simulink model "Cyber_Physical_Microgrid"  (R2024b)
settings: Solver=VariableStepAuto  StartTime=0.0  StopTime=270  RelTol=1e-3
values from neighbouring files (symbols this model uses):
  Bat =     [initData.mat]
  droopFC1 = 0.05    [initData.mat]
  droopFC2 = 0.05    [initData.mat]
  droopP2 = 0.05    [initData.mat]
  droopQ1 = 0.05    [initData.mat]
  droopQ2 = 0.05    [initData.mat]
  Pref2 = 0.8    [initData.mat]
  Qref1 = 0    [initData.mat]
  Qref2 = 0    [initData.mat]
  timeACLoadCurtail = 200    [initData.mat]
  timeSolarCurtail = 200    [initData.mat]
  Ts = 5e-05    [initData.mat]
  Ts_AC = 0.0002    [initData.mat]
  Ts_DC = 0.001    [initData.mat]
  volt2 = [270.467186401 250.166401688 246.278575679 243.847178474 242.073246789 240.654489675 239.457734124 238.414696845 237.485238449 236.643553985 235.871256975 235.151075236 ... (161 elements, 1x161)]    [initData.mat]
undefined symbols (not defined in the file or in its folder): BattTempBp, CapLUTBp, CapSOCBp, DiscIntNeverNeededParam, Em, Np, Ns, RInt, Tc_Batt
libraries: nesl_utility x55, fl_lib x52, ee_lib x39, modbuslib x16, spsRMSLib x8, simulink x5, spsFourierLib x2, batteryecm_lib x1, eeTransforms x1
(part 2 of 3)

== system Cyber_Physical_Microgrid/Grid Synchronization ==
  note: breaker command: 1 - islanded (PCC open)
      | 0 - connect to utility (PCC closed)
  note: 1 - start sycnhronisation
      | 0 - stay islanded
  note: microgrid frequency (pu)
  note: utility grid phase angle
  note: microgrid phase angle
  note: new frequency reference sent to
      | microgrid governer
  note: utility grid frequency (pu)
  note: frequency step size (how aggressive we tune frequency)
  Constant1 : Constant  Value=1e-5
  Constant2 : Constant
  Grid Synchronization1 : MATLAB Function  TreatAsAtomicUnit=on
  Step : Step  Time=27  Before=1  After=0  SampleTime=0
  Unit Delay : UnitDelay  InitialCondition=1  SampleTime=Ts_AC  HasFrameUpgradeWarning=on
  Unit Delay1 : UnitDelay  InitialCondition=1  SampleTime=Ts_AC  HasFrameUpgradeWarning=on
  tag scope: freqRef=global, gridEnable=global, synchStart=global
  wires:
  Grid Synchronization1/2(gridEnable) -> Unit Delay/1  "gridEnable"
  Constant1/1 -> Grid Synchronization1/1(deltaF)
  [phiMicro] -> Grid Synchronization1/5(phiMicro)
  Unit Delay1/1 -> [freqRef]
  [freq_gen1_pu] -> Grid Synchronization1/3(freqMicro)
  Grid Synchronization1/1(freqRef) -> Unit Delay1/1
  Constant2/1 -> Grid Synchronization1/2(freqUtility)
  Unit Delay/1 -> [gridEnable]
  [phiUtility] -> Grid Synchronization1/4(phiUtility)
  Step/1 -> [synchStart], Grid Synchronization1/6(synchStart)

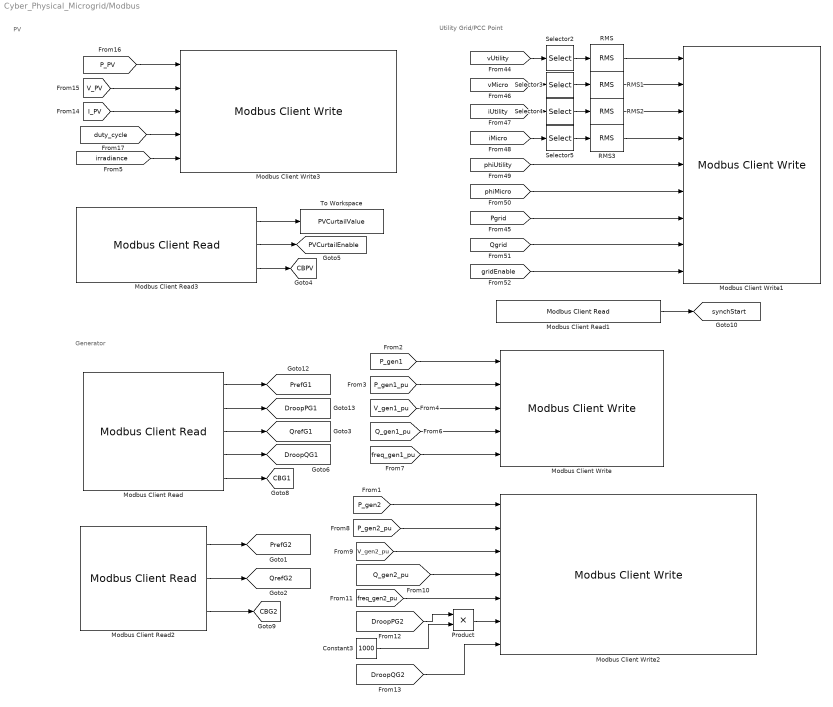
== system Cyber_Physical_Microgrid/Modbus ==
  note: PV
  note: Utility Grid/PCC Point
  note: Generator
  Constant3 : Constant  Value=1000
  Modbus Client Read : modbuslib/Modbus Client Read  RetainClient=gen1  ClientList=gen1  ConnectionEndpoint=192.168.1.202:502  ServerId=1  RegisterTable={ '1', 'PrefG1', '21', 'Holding Register', 'double', '1'; '2', 'DroopPG1', '25', 'Holding Register', 'double', '1'; '3', 'QrefG1', '29', 'Holding Register', 'double', '1'; '4', 'DroopQG1', '34', 'Holding Register', 'double', '1'; '5', 'CBG1', '38', 'Coil', 'bit', '1' }  SampleTime=1
  Modbus Client Read1 : modbuslib/Modbus Client Read  RetainClient=ModbusClient  ClientList=ModbusClient  ConnectionEndpoint=192.168.1.201:502  ServerId=1  RegisterTable={ '1', 'synchStart', '38', 'Coil', 'bit', '1' }  SampleTime=1
  Modbus Client Read2 : modbuslib/Modbus Client Read  RetainClient=gen2  ClientList=gen2  ConnectionEndpoint=192.168.1.203:502  ServerId=1  RegisterTable={ '1', 'PrefG2', '21', 'Holding Register', 'double', '1'; '2', 'QrefG2', '29', 'Holding Register', 'double', '1'; '3', 'CBG2', '38', 'Coil', 'bit', '1' }  SampleTime=1
  Modbus Client Read3 : modbuslib/Modbus Client Read  RetainClient=pv  ClientList=pv  ConnectionEndpoint=192.168.1.204:502  ServerId=1  RegisterTable={ '1', 'PvCurtailValue', '21', 'Holding Register', 'double', '1'; '2', 'curtail enable', '25', 'Coil', 'bit', '1'; '3', 'CBPV', '29', 'Coil', 'bit', '1' }  SampleTime=1
  Modbus Client Write : modbuslib/Modbus Client Write  RetainClient=gen1  ClientList=gen1  ConnectionEndpoint=192.168.1.202:502  ServerId=1  RegisterTable={ '1', 'P_gen1', '1', 'Holding Register', 'double'; '2', 'P_gen1_pu', '5', 'Holding Register', 'double'; '3', 'V_gen1_pu', '9', 'Holding Register', 'double'; '4', 'Q_gen1_pu', '13', 'Holding Register', 'double'; '5', 'freq_gen1_pu', '17', 'Holding Register', 'double' }  SampleTime=1
  Modbus Client Write1 : modbuslib/Modbus Client Write  RetainClient=ModbusClient  ClientList=ModbusClient  ConnectionEndpoint=192.168.1.201:502  ServerId=1  RegisterTable={ '1', 'vUtility_rms', '1', 'Holding Register', 'double'; '2', 'vMicro_rms', '5', 'Holding Register', 'double'; '3', 'iUtility_rms', '9', 'Holding Register', 'double'; '4', 'iMicro_rms', '13', 'Holding Register', 'double'; '5', 'phiUtility', '17', 'Holding Register', 'double'; '6', 'phiMicro', '21', 'Holding Register', 'double'; '7', 'Pgrid', '25', 'Holding Register', 'double'; '8', 'Qgrid', '29', 'Holding Register', 'double'; '9', 'gridEnable', '34', 'Coil', 'bit' }  SampleTime=1
  Modbus Client Write2 : modbuslib/Modbus Client Write  RetainClient=gen2  ClientList=gen2  ConnectionEndpoint=192.168.1.203:502  ServerId=1  RegisterTable={ '1', 'P_gen2', '1', 'Holding Register', 'double'; '2', 'P_gen2_pu', '5', 'Holding Register', 'double'; '3', 'V_gen2_pu', '9', 'Holding Register', 'double'; '4', 'Q_gen2_pu', '13', 'Holding Register', 'double'; '5', 'freq_gen2_pu', '17', 'Holding Register', 'double'; '6', 'DroopPG2', '25', 'Holding Register', 'double'; '7', 'DroopQG2', '34', 'Holding Register', 'double' }  SampleTime=1
  Modbus Client Write3 : modbuslib/Modbus Client Write  RetainClient=pv  ClientList=pv  ConnectionEndpoint=192.168.1.204:502  ServerId=1  RegisterTable={ '1', 'P_PV', '1', 'Holding Register', 'double'; '2', 'V_PV', '5', 'Holding Register', 'double'; '3', 'I_PV', '9', 'Holding Register', 'double'; '4', 'duty cycle', '13', 'Holding Register', 'double'; '5', 'irradiance', '17', 'Holding Register', 'double' }  SampleTime=1
  Product : Product
  RMS{,1..3} (4 alike) : spsRMSLib/RMS  TrueRMS=on  Freq=50  RMSInit=120  Ts=0
  Selector{2..5} (4 alike) : Selector  InputPortWidth=3  IndexOptions=Index vector (dialog)  Indices=1  OutputSizes=1
  To Workspace : ToWorkspace  VariableName=PVCurtailValue  SaveFormat=Timeseries  SampleTime=-1
  tag scope: CBG1=global, CBG2=global, CBPV=global, DroopPG1=global, DroopQG1=global, PVCurtailEnable=global, PrefG1=global, PrefG2=global, QrefG1=global, QrefG2=global, synchStart=global
  wires:
  [V_gen1_pu] -> Modbus Client Write/3
  [P_gen1_pu] -> Modbus Client Write/2
  Modbus Client Read/1 -> [PrefG1]
  [P_gen1] -> Modbus Client Write/1
  [freq_gen1_pu] -> Modbus Client Write/5
  [Q_gen1_pu] -> Modbus Client Write/4
  Modbus Client Read/2 -> [DroopPG1]
  Modbus Client Read/5 -> [CBG1]
  [iMicro] -> Selector5/1
  RMS2/1 -> Modbus Client Write1/3
  RMS/1 -> Modbus Client Write1/1
  RMS3/1 -> Modbus Client Write1/4
  [iUtility] -> Selector4/1
  [phiUtility] -> Modbus Client Write1/5
  [Qgrid] -> Modbus Client Write1/8
  [Pgrid] -> Modbus Client Write1/7
  Selector4/1 -> RMS2/1
  Selector5/1 -> RMS3/1
  RMS1/1 -> Modbus Client Write1/2
  Modbus Client Read1/1 -> [synchStart]
  [vMicro] -> Selector3/1
  [vUtility] -> Selector2/1
  [phiMicro] -> Modbus Client Write1/6
  [gridEnable] -> Modbus Client Write1/9
  Selector2/1 -> RMS/1
  Selector3/1 -> RMS1/1
  Constant3/1 -> Product/2
  [P_gen2] -> Modbus Client Write2/1
  [DroopPG2] -> Product/1
  [V_gen2_pu] -> Modbus Client Write2/3
  Product/1 -> Modbus Client Write2/6
  Modbus Client Read2/3 -> [CBG2]
  Modbus Client Read2/2 -> [QrefG2]
  [DroopQG2] -> Modbus Client Write2/7
  [freq_gen2_pu] -> Modbus Client Write2/5
  [Q_gen2_pu] -> Modbus Client Write2/4
  [P_gen2_pu] -> Modbus Client Write2/2
  Modbus Client Read2/1 -> [PrefG2]
  Modbus Client Read3/3 -> [CBPV]
  [P_PV] -> Modbus Client Write3/1
  Modbus Client Read3/1 -> To Workspace/1
  [irradiance] -> Modbus Client Write3/5
  [duty_cycle] -> Modbus Client Write3/4
  [I_PV] -> Modbus Client Write3/3
  Modbus Client Read3/2 -> [PVCurtailEnable]
  [V_PV] -> Modbus Client Write3/2
  Modbus Client Read/3 -> [QrefG1]
  Modbus Client Read/4 -> [DroopQG1]

== system Cyber_Physical_Microgrid/PQ meas ==
  PS-Simulink Converter : nesl_utility/PS-Simulink Converter  PhysicalDomain=network_engine_domain  SubClassName=ps_output  LeftPortType=input  RightPortType=output  PseudoPeriodic=off  Frequencies=[]  VectorFormat=1-D array  Unit=W  AffineConversion=off
  PS-Simulink Converter1 : nesl_utility/PS-Simulink Converter  PhysicalDomain=network_engine_domain  SubClassName=ps_output  LeftPortType=input  RightPortType=output  PseudoPeriodic=off  Frequencies=[]  VectorFormat=1-D array  Unit=V*A  AffineConversion=off
  Power Sensor (Three-Phase) : ee_lib/Sensors & Transducers/Power Sensor (Three-Phase)  load_type=ee.enum.passive.type_balanced.balanced  f0=50 Hz
      settings: InternalSimscapePortConfiguration="{\"Bottom\":[],\"Left\":[{\"id\":\"N1\",\"label\":\"~1\",\"type\":\"foundation.electrical.three_phase\"}],\"Right\":[{\"id\":\"N2\",\"label\":\"~2\",\"type\":\"foundation.electrical.three_phase\"}],\"Top\":[{\"id\":\"Pm\",\"label\":\"P\",\"type\":\"output\"},{\"id\":\"Qm\",\"label\":\"Q\",\"type\":\"output\"}]}"
  Subsystem : Subsystem
  Subsystem1 : Subsystem
  ~1 : PMIOPort  Side=Left
  ~2 : PMIOPort  Port=2  Side=Right
  tag scope: P_load=global, Q_load=global
  wires:
  PS-Simulink Converter1/1 -> Subsystem1/1(In1)
  Subsystem1/1(Out1) -> [Q_load]  "Q_load"
  Subsystem/1(Out1) -> [P_load]  "P_load"
  PS-Simulink Converter/1 -> Subsystem/1(In1)
  connections:
  ~2/RConn1 -- Power Sensor (Three-Phase)/RConn1
  Power Sensor (Three-Phase)/LConn1 -- ~1/RConn1
  PS-Simulink Converter/LConn1 -- Power Sensor (Three-Phase)/LConn2
  PS-Simulink Converter1/LConn1 -- Power Sensor (Three-Phase)/LConn3

== system Cyber_Physical_Microgrid/PV Array ==
  Display : Display
  ERef : fl_lib/Electrical/Electrical Elements/Electrical Reference
  Product1 : Product
  Repeating Sequence Interpolated : simulink/Sources/Repeating Sequence Interpolated  OutValues=[1e-3 1e-3 1 1]*1000  TimeValues=[0 1 5 300]  LookUpMeth=Interpolation-Use End Values  tsamp=Ts_DC  OutMin=[]  OutMax=[]  OutDataTypeStr=double  OutputDataTypeScalingMode=double  OutDataType=fixdt(0,8)  OutScaling=2^-10
  Sensing Current : Subsystem
      settings: PortSchema="{\"entries\":[{\"content\":{\"sides\":[{\"content\":{\"connectorIds\":[\"LConn1\"]},\"type\":\"ConnectorPlacement.EquallySpacedRectSide\",\"uuid\":\"08eaf192-3836-4d70-9f6a-c3aee0977ea6\"},{\"content\":{\"connectorIds\":[\"RConn1\"],\"side\":\"RIGHT\"},\"type\":\"ConnectorPlacement.EquallySpacedRectSide\",\"uuid\":\"69615d36-c1bf-4d31-b3e4-77c73286e7c7\"},{\"content\":{\"connectorIds\":[\"Out1\"],\"side\":\"TOP\"},\"type\":\"ConnectorPlacement.EquallySpacedRectSide\",\"uuid\":\"21e31d90-f675-47e5-98f5-1bf7e6a5fdbe\"}]},\"type\":\"ConnectorPlacement.EquallySpacedConnector\",\"uuid\":\"068abd2e-abc9-41d7-b40e-d83d3e3b9346\"}],\"packageUris\":[\"http://schema.mathworks.com/mf0/Connector/R2020b\"],\"version\":\"1.0\"}"
      mask Display: disp('i')
  Simulink-PS Converter : nesl_utility/Simulink-PS Converter  PhysicalDomain=network_engine_domain  SubClassName=ps_input  LeftPortType=input  RightPortType=output  PseudoPeriodic=off  Frequencies=[]  NoiseDistribution=none  NoiseParameters=[]  Unit=1  AffineConversion=off  FilteringAndDerivatives=provide  SimscapeFilterOrder=1  InputFilterTimeConstant=0.001  UdotUserProvided=0
  Solar Cell : ee_lib/Sources/Solar Cell  PartSpecification="{\"DatasetId\":\"Amerisolar|AS_6M30_HC_320W|simscape.electrical.solarCell\",\"DisplayName\":\"Amerisolar:AS_6M30_HC_320W\"}"  prm=3  Isc=10.14 A  Voc=0.67 V  Is=3.24823447983853e-07 A  Is2=9.37081970792037e-10 A  Iph=10.140005507508 A  Ir0=1000 W/m^2  ec=1.51118472243322  N2=2.60259908345858  Rs=1.94548269975201e-05 Ohm  Rp=682.95993142779 Ohm  N_series=60*100  N_parallel=30  TIPH1=0.000499942933005141 1/K  EG=1.12 eV  TXIS1=4.23641510120988  TXIS2=16.2689137700667  TRS1=0.243341028305912  TRP1=0 % Parameter not set  Tmeas=25 degC  TFIXED=30 degC  thermal_mass=100 % Parameter not set J/K  initial_temperature=25 degC
      settings: AttributesFormatString=Amerisolar:AS_6M30_HC_320W
  Terminator : Terminator
  sensing voltage : Subsystem
      settings: PortSchema="{\"entries\":[{\"content\":{\"sides\":[{\"content\":{\"connectorIds\":[\"LConn1\"]},\"type\":\"ConnectorPlacement.EquallySpacedRectSide\",\"uuid\":\"08eaf192-3836-4d70-9f6a-c3aee0977ea6\"},{\"content\":{\"connectorIds\":[\"RConn1\"],\"side\":\"RIGHT\"},\"type\":\"ConnectorPlacement.EquallySpacedRectSide\",\"uuid\":\"69615d36-c1bf-4d31-b3e4-77c73286e7c7\"},{\"content\":{\"connectorIds\":[],\"side\":\"TOP\"},\"type\":\"ConnectorPlacement.EquallySpacedRectSide\",\"uuid\":\"21e31d90-f675-47e5-98f5-1bf7e6a5fdbe\"},{\"content\":{\"connectorIds\":[\"Out1\"],\"side\":\"BOTTOM\"},\"type\":\"ConnectorPlacement.EquallySpacedRectSide\",\"uuid\":\"23a77980-6beb-4147-b48e-adf9e1983263\"}]},\"type\":\"ConnectorPlacement.EquallySpacedConnector\",\"uuid\":\"068abd2e-abc9-41d7-b40e-d83d3e3b9346\"}],\"packageUris\":[\"http://schema.mathworks.com/mf0/Connector/R2020b\"],\"version\":\"1.0\"}"
      mask Display: disp('v')
  - : PMIOPort  Side=Left
  -1 : PMIOPort  Port=2  Side=Left
  tag scope: I_PV=global, V_PV=global, irradiance=global
  wires:
  sensing voltage/1(V) -> Display/1, [V_PV], Product1/2  "V_PV"
  Product1/1 -> Terminator/1  "P_PV"
  Repeating Sequence Interpolated/1 -> [irradiance], Simulink-PS Converter/1  "irradiance"
  Sensing Current/1(I) -> [I_PV], Product1/1  "I_PV"
  connections:
  Solar Cell/LConn1 -- Simulink-PS Converter/RConn1
  Solar Cell/LConn2 -- Sensing Current/LConn1
  sensing voltage/RConn1 -- Solar Cell/RConn1 -- ERef/LConn1 -- -1/RConn1
  sensing voltage/LConn1 -- -/RConn1 -- Sensing Current/RConn1

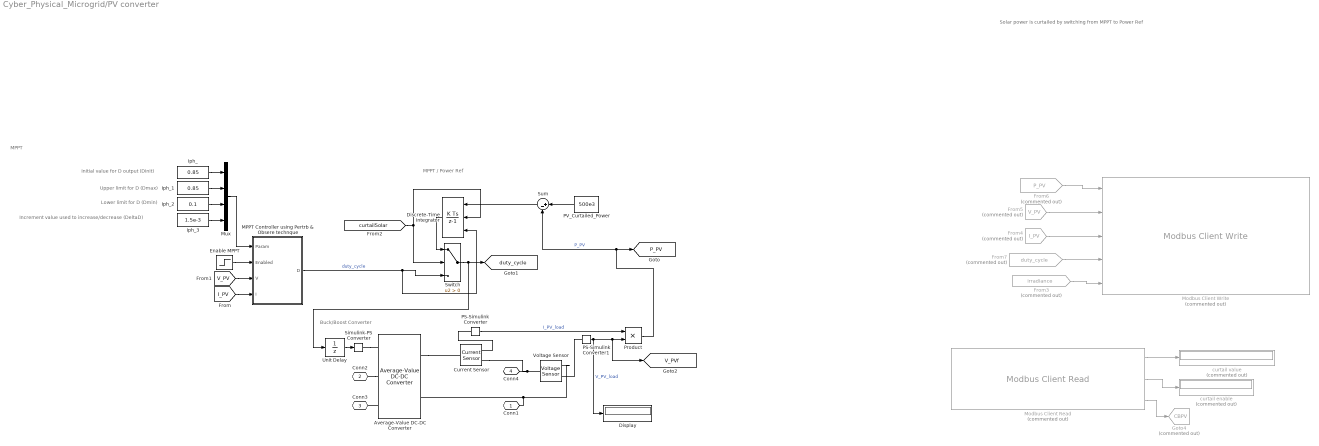
== system Cyber_Physical_Microgrid/PV converter ==
  note: Lower limit for D (Dmin)
  note: Upper limit for D (Dmax)
  note: Increment value used to increase/decrease (DeltaD)
  note: Initial value for D output (Dinit)
  note: Solar power is curtailed by switching from MPPT to Power Ref
  note: MPPT / Power Ref
  note: MPPT
  note: Buck/Boost Converter
  Average-Value DC-DC Converter : ee_lib/Semiconductors & Converters/Converters/Average-Value DC-DC Converter  control_option=ee.enum.converters.controlinput.dutycycle  converter_type=ee.enum.converters.dcdctype.buckboost  efficiency_option=ee.enum.converters.efficiency.constant  efficiency_fixed=100  i_vec=[0, 2, 5] A  efficiency_vec=[90, 95, 98]
      settings: InternalSimscapePortConfiguration="{\"Bottom\":[],\"Left\":[{\"id\":\"DutyCycle\",\"label\":\"DutyCycle\",\"type\":\"input\"},{\"id\":\"p1\",\"label\":\"1+\",\"type\":\"foundation.electrical.electrical\"},{\"id\":\"n1\",\"label\":\"1-\",\"type\":\"foundation.electrical.electrical\"}],\"Right\":[{\"id\":\"p2\",\"label\":\"2+\",\"type\":\"foundation.electrical.electrical\"},{\"id\":\"n2\",\"label\":\"2-\",\"type\":\"foundation.electrical.electrical\"}],\"Top\":[]}"
  Current Sensor : fl_lib/Electrical/Electrical Sensors/Current Sensor
  Discrete-Time Integrator : DiscreteIntegrator  gainval=1e-6  ExternalReset=rising  InitialConditionSource=external  SampleTime=-1  ICPrevOutput=DiscIntNeverNeededParam  ICPrevScaledInput=DiscIntNeverNeededParam
  Display : Display
  Enable MPPT : Step  Time=0.1  SampleTime=Ts_DC
  From3 : From  Commented=on  GotoTag=irradiance  TagVisibility=global
  From4 : From  Commented=on  GotoTag=I_PV  TagVisibility=global
  From5 : From  Commented=on  GotoTag=V_PV  TagVisibility=global
  From6 : From  Commented=on  GotoTag=P_PV  TagVisibility=global
  From7 : From  Commented=on  GotoTag=duty_cycle  TagVisibility=global
  Goto4 : Goto  Commented=on  GotoTag=CBPV  TagVisibility=global
  Iph_ : Constant  Value=0.85  SampleTime=Ts_DC
  Iph_1 : Constant  Value=0.85  SampleTime=Ts_DC
  Iph_2 : Constant  Value=0.1  SampleTime=Ts_DC
  Iph_3 : Constant  Value=1.5e-3  SampleTime=Ts_DC
  "MPPT Controller using Pertrb & Obsere technque " : MATLAB Function  SystemSampleTime=Ts
  Modbus Client Read : modbuslib/Modbus Client Read  Commented=on  RetainClient=No Modbus client available  ClientList=No Modbus client available  ConnectionEndpoint=No Modbus client selected  ServerId=1  RegisterTable={ '1', 'PvCurtailValue', '21', 'Holding Register', 'double', '1'; '2', 'curtail enable', '25', 'Coil', 'bit', '1'; '3', 'CBPV', '29', 'Coil', 'bit', '1' }  SampleTime=1
  Modbus Client Write : modbuslib/Modbus Client Write  Commented=on  RetainClient=No Modbus client available  ClientList=No Modbus client available  ConnectionEndpoint=No Modbus client selected  ServerId=1  RegisterTable={ '1', 'P_PV', '1', 'Holding Register', 'double'; '2', 'V_PV', '5', 'Holding Register', 'double'; '3', 'I_PV', '9', 'Holding Register', 'double'; '4', 'duty cycle', '13', 'Holding Register', 'double'; '5', 'irradiance', '17', 'Holding Register', 'double' }  SampleTime=1
  Mux : Mux
  PS-Simulink Converter : nesl_utility/PS-Simulink Converter  PhysicalDomain=network_engine_domain  SubClassName=ps_output  LeftPortType=input  RightPortType=output  PseudoPeriodic=off  Frequencies=[]  VectorFormat=1-D array  Unit=inherit  AffineConversion=off
  PS-Simulink Converter1 : nesl_utility/PS-Simulink Converter  PhysicalDomain=network_engine_domain  SubClassName=ps_output  LeftPortType=input  RightPortType=output  PseudoPeriodic=off  Frequencies=[]  VectorFormat=1-D array  Unit=inherit  AffineConversion=off
  PV_Curtailed_Power : Constant  Value=500e3
  Product : Product
  Simulink-PS Converter : nesl_utility/Simulink-PS Converter  PhysicalDomain=network_engine_domain  SubClassName=ps_input  LeftPortType=input  RightPortType=output  PseudoPeriodic=off  Frequencies=[]  NoiseDistribution=none  NoiseParameters=[]  Unit=1  AffineConversion=off  FilteringAndDerivatives=provide  SimscapeFilterOrder=1  InputFilterTimeConstant=0.001  UdotUserProvided=0
  Sum : Sum  Inputs=|+-
  Switch : Switch  Criteria=u2 > Threshold  SaturateOnIntegerOverflow=off  InputSameDT=off
  Unit Delay : UnitDelay  InitialCondition=0.99  SampleTime=-1  HasFrameUpgradeWarning=on
  Voltage Sensor : fl_lib/Electrical/Electrical Sensors/Voltage Sensor
  curtail enable : Display  Commented=on
      settings: Format=decimal (Stored Integer)  Decimation=4
  curtail value : Display  Commented=on
      settings: Format=decimal (Stored Integer)  Decimation=4
  Conn1 : PMIOPort  Side=Left
  Conn2 : PMIOPort  Port=2  Side=Left
  Conn3 : PMIOPort  Port=3  Side=Left
  Conn4 : PMIOPort  Port=4  Side=Left
  tag scope: P_PV=global, V_PVf=global, duty_cycle=global
  wires:
  From7/1 -> Modbus Client Write/4
  Enable MPPT/1 -> "MPPT Controller using Pertrb & Obsere technque "/2(Enabled)
  Modbus Client Read/2 -> curtail enable/1
  Iph_1/1 -> Mux/2
  Mux/1 -> "MPPT Controller using Pertrb & Obsere technque "/1(Param)
  [V_PV] -> "MPPT Controller using Pertrb & Obsere technque "/3(V)
  Unit Delay/1 -> Simulink-PS Converter/1
  From4/1 -> Modbus Client Write/3
  Iph_2/1 -> Mux/3
  PS-Simulink Converter1/1 -> Display/1, [V_PVf], Product/2  "V_PV_load"
  [curtailSolar] -> Discrete-Time Integrator/2, Switch/2
  Iph_/1 -> Mux/1
  From5/1 -> Modbus Client Write/2
  PS-Simulink Converter/1 -> Product/1  "I_PV_load"
  Iph_3/1 -> Mux/4
  From6/1 -> Modbus Client Write/1
  Sum/1 -> Discrete-Time Integrator/1
  Modbus Client Read/3 -> Goto4/1
  "MPPT Controller using Pertrb & Obsere technque "/1(D) -> Discrete-Time Integrator/3, Switch/3  "duty_cycle"
  PV_Curtailed_Power/1 -> Sum/1
  Modbus Client Read/1 -> curtail value/1
  Product/1 -> Sum/2, [P_PV]  "P_PV"
  From3/1 -> Modbus Client Write/5
  [I_PV] -> "MPPT Controller using Pertrb & Obsere technque "/4(I)
  Discrete-Time Integrator/1 -> Switch/1
  Switch/1 -> Unit Delay/1, [duty_cycle]
  connections:
  Conn2/RConn1 -- Average-Value DC-DC Converter/LConn2
  Current Sensor/RConn2 -- Voltage Sensor/LConn1 -- Conn4/RConn1
  Simulink-PS Converter/RConn1 -- Average-Value DC-DC Converter/LConn1
  Average-Value DC-DC Converter/RConn1 -- Current Sensor/LConn1
  Voltage Sensor/RConn2 -- Conn1/RConn1 -- Average-Value DC-DC Converter/RConn2
  PS-Simulink Converter/LConn1 -- Current Sensor/RConn1
  Average-Value DC-DC Converter/LConn3 -- Conn3/RConn1
  PS-Simulink Converter1/LConn1 -- Voltage Sensor/RConn1

== system Cyber_Physical_Microgrid/Power Converter ==
  AC/DC Power Conversion : Subsystem
      settings: PortSchema="{\"entries\":[{\"content\":{\"sides\":[{\"content\":{\"connectorIds\":[\"LConn1\"]},\"type\":\"ConnectorPlacement.EquallySpacedRectSide\",\"uuid\":\"019ca52f-1b20-4f8a-8000-26047d27ba44\"},{\"content\":{\"connectorIds\":[\"RConn1\",\"RConn2\"],\"side\":\"RIGHT\"},\"type\":\"ConnectorPlacement.EquallySpacedRectSide\",\"uuid\":\"bc0710a3-2fa6-4c07-a357-204360cbd971\"},{\"content\":{\"connectorIds\":[\"In1\",\"In2\"],\"side\":\"TOP\"},\"type\":\"ConnectorPlacement.EquallySpacedRectSide\",\"uuid\":\"62c22250-eba7-4d66-a03a-98d0551949f6\"}]},\"type\":\"ConnectorPlacement.EquallySpacedConnector\",\"uuid\":\"4a6536c9-62d3-4a93-9f4d-cdcce83d66f7\"}],\"packageUris\":[\"http://schema.mathworks.com/mf0/Connector/R2020b\"],\"version\":\"1.0\"}"
      mask Display: disp('Ideal AC/DC\nPower Conversion')
  Current Sensor : fl_lib/Electrical/Electrical Sensors/Current Sensor
  Display : Display
  Electrical Reference : fl_lib/Electrical/Electrical Elements/Electrical Reference
  PS-Simulink Converter : nesl_utility/PS-Simulink Converter  PhysicalDomain=network_engine_domain  SubClassName=ps_output  LeftPortType=input  RightPortType=output  PseudoPeriodic=off  Frequencies=[]  VectorFormat=inherit  Unit=inherit  AffineConversion=off
  PS-Simulink Converter1 : nesl_utility/PS-Simulink Converter  PhysicalDomain=network_engine_domain  SubClassName=ps_output  LeftPortType=input  RightPortType=output  PseudoPeriodic=off  Frequencies=[]  VectorFormat=inherit  Unit=inherit  AffineConversion=off
  Product : Product
  Qref : simulink/Sources/Repeating Sequence Interpolated  OutValues=[0 0 0 0]*1e5  TimeValues=[0 11 13 50]  LookUpMeth=Interpolation-Use End Values  tsamp=Ts_AC  OutMin=[]  OutMax=[]  OutDataTypeStr=double  OutputDataTypeScalingMode=double  OutDataType=fixdt(0,8)  OutScaling=2^-10
  Solver Configuration : nesl_utility/Solver Configuration  PhysicalDomain=network_engine_domain  SubClassName=solver  LeftPortType=input  RightPortType=generic  Tones=[]  Harmonics=[]  SimulateNoise=off  Profile=off  UseLocalSampling=off  EnableSwitchedLinearOptims=on  FrequencyDomain=off  UseCCode=off  RelTol=0.001  AbsTol=1e-06  MinStep=1e-09  ToWorkspace=off  RevertToSquareIcSolve=off  NumHomotopyIterations=100  PhasorMode=off  PhasorModeNumHarmonics=1  ConsistencySolver=NEWTON_FTOL  IndexReductionMethod=DerivativeReplacement  DoDC=off  ResidualTolerance=1e-09  ConsistencyTolSource=GLOBAL  ConsistencyAbsTol=0.001  ConsistencyRelTol=0.001  ConsistencyTolFactor=0.001  UseLocalSolver=on  LocalSolverChoice=NE_PARTITIONING_ADVANCER  ResolveIndetEquations=on  FunctionEvalNumThread=1  LocalSolverSampleTime=Ts_DC  DoFixedCost=on  MaxNonlinIter=1  MaxModeIter=2  ComputeImpulses=off  ImpulseIterations=2  LinearAlgebra=auto  LinearAlgebraNumThread=0  EquationFormulation=NE_TIME_EF  DelaysMemoryBudget=1024  AutomaticFiltering=on  FilteringTimeConstant=0.001  PartitionStorageMethod=AS_NEEDED  PartitionMemoryBudget=1024  PartitionMethod=ROBUST  MultibodyUseLocalSolver=off  MultibodyLocalSolverChoice=ODE1  MultibodyLocalSolverSampleTime=0.001
  Voltage Sensor : fl_lib/Electrical/Electrical Sensors/Voltage Sensor
  ~ : PMIOPort  Side=Left
  + : PMIOPort  Port=2  Side=Right
  - : PMIOPort  Port=3  Side=Right
  wires:
  Qref/1 -> AC/DC Power Conversion/2(Qref)
  [P_AC_ref] -> AC/DC Power Conversion/1(Pref)
  PS-Simulink Converter1/1 -> Product/2
  PS-Simulink Converter/1 -> Product/1
  Product/1 -> Display/1
  connections:
  AC/DC Power Conversion/LConn1 -- ~/RConn1
  Current Sensor/LConn1 -- Voltage Sensor/LConn1 -- AC/DC Power Conversion/RConn1
  AC/DC Power Conversion/RConn2 -- -/RConn1 -- Voltage Sensor/RConn2 -- Electrical Reference/LConn1
  Solver Configuration/RConn1 -- +/RConn1 -- Current Sensor/RConn2
  PS-Simulink Converter/LConn1 -- Current Sensor/RConn1
  PS-Simulink Converter1/LConn1 -- Voltage Sensor/RConn1

== system Cyber_Physical_Microgrid/Reactive Power Load ==
  Electrical Reference1 : fl_lib/Electrical/Electrical Elements/Electrical Reference
  PS Divide : fl_lib/Physical Signals/Functions/PS Divide
  PS Product : fl_lib/Physical Signals/Functions/PS Product
  Phase Splitter1 : ee_lib/Connectors & References/Phase Splitter
  Reactive Power Reference : simulink/Sources/Repeating Sequence Interpolated  OutValues=[1e-6 1e-6 1e-6]*6e6*2*pi*50  TimeValues=[0 1 50]  LookUpMeth=Interpolation-Use End Values  tsamp=Ts_AC  OutMin=[]  OutMax=[]  OutDataTypeStr=double  OutputDataTypeScalingMode=double  OutDataType=fixdt(0,8)  OutScaling=2^-10
  Simulink-PS Converter1 : nesl_utility/Simulink-PS Converter  PhysicalDomain=network_engine_domain  SubClassName=ps_input  LeftPortType=input  RightPortType=output  PseudoPeriodic=off  Frequencies=[]  NoiseDistribution=none  NoiseParameters=[]  Unit=V*A*rad/s  AffineConversion=off  FilteringAndDerivatives=provide  SimscapeFilterOrder=1  InputFilterTimeConstant=0.001  UdotUserProvided=0
  Variable Inductor : ee_lib/Passive/Variable Inductor  prm=2  Lmin=1e-6 H  g=0 1/Ohm  i0=0 A  phi0=0 Wb
      settings: InternalSimscapePortConfiguration="{\"Bottom\":[],\"Left\":[{\"id\":\"L\",\"label\":\"L\",\"type\":\"input\"},{\"id\":\"p\",\"label\":\"+\",\"type\":\"foundation.electrical.electrical\"}],\"Right\":[{\"id\":\"n\",\"label\":\"-\",\"type\":\"foundation.electrical.electrical\"}],\"Top\":[]}"
  Variable Inductor1 : ee_lib/Passive/Variable Inductor  prm=2  Lmin=1e-6 H  g=0 1/Ohm  i0=0 A  phi0=0 Wb
      settings: InternalSimscapePortConfiguration="{\"Bottom\":[],\"Left\":[{\"id\":\"L\",\"label\":\"L\",\"type\":\"input\"},{\"id\":\"p\",\"label\":\"+\",\"type\":\"foundation.electrical.electrical\"}],\"Right\":[{\"id\":\"n\",\"label\":\"-\",\"type\":\"foundation.electrical.electrical\"}],\"Top\":[]}"
  Variable Inductor2 : ee_lib/Passive/Variable Inductor  prm=2  Lmin=1e-6 H  g=0 1/Ohm  i0=0 A  phi0=0 Wb
      settings: InternalSimscapePortConfiguration="{\"Bottom\":[],\"Left\":[{\"id\":\"L\",\"label\":\"L\",\"type\":\"input\"},{\"id\":\"p\",\"label\":\"+\",\"type\":\"foundation.electrical.electrical\"}],\"Right\":[{\"id\":\"n\",\"label\":\"-\",\"type\":\"foundation.electrical.electrical\"}],\"Top\":[]}"
  Vnom : fl_lib/Physical Signals/Sources/PS Constant  constant=6600*0.98 V
  Conn1 : PMIOPort  Side=Left
  wires:
  Reactive Power Reference/1 -> Simulink-PS Converter1/1
  connections:
  Phase Splitter1/RConn3 -- Variable Inductor2/LConn2
  PS Product/LConn2 -- PS Product/LConn1 -- Vnom/RConn1
  PS Divide/LConn1 -- PS Product/RConn1
  Simulink-PS Converter1/RConn1 -- PS Divide/LConn2
  Variable Inductor/LConn1 -- Variable Inductor2/LConn1 -- Variable Inductor1/LConn1 -- PS Divide/RConn1
  Variable Inductor1/LConn2 -- Phase Splitter1/RConn2
  Variable Inductor/RConn1 -- Variable Inductor1/RConn1 -- Variable Inductor2/RConn1 -- Electrical Reference1/LConn1
  Phase Splitter1/RConn1 -- Variable Inductor/LConn2
  Phase Splitter1/LConn1 -- Conn1/RConn1

== system Cyber_Physical_Microgrid/Subsystem ==
  Circuit Breaker at GEN1 : ee_lib/Switches & Breakers/Circuit Breaker (Three-Phase)  R_closed=1e-6 Ohm  G_open=1e-6 1/Ohm  threshold=0.5 V  breaker_behavior=ee.enum.switches.breakerBehavior.zeroCrossingEnable
      settings: InternalSimscapePortConfiguration="{\"Bottom\":[],\"Left\":[{\"id\":\"vT\",\"label\":\"vT\",\"type\":\"input\"},{\"id\":\"N1\",\"label\":\"~1\",\"type\":\"foundation.electrical.three_phase\"}],\"Right\":[{\"id\":\"N2\",\"label\":\"~2\",\"type\":\"foundation.electrical.three_phase\"}],\"Top\":[]}"
  Conn1 : PMIOPort  Side=Right
  Conn2 : PMIOPort  Port=2  Side=Left
  Conn3 : PMIOPort  Port=3  Side=Left
  connections:
  Conn3/RConn1 -- Circuit Breaker at GEN1/LConn1
  Circuit Breaker at GEN1/RConn1 -- Conn1/RConn1
  Conn2/RConn1 -- Circuit Breaker at GEN1/LConn2

== system Cyber_Physical_Microgrid/Subsystem1 ==
  Circuit Breaker at GEN2 : ee_lib/Switches & Breakers/Circuit Breaker (Three-Phase)  R_closed=1e-6 Ohm  G_open=1e-6 1/Ohm  threshold=0.5 V  breaker_behavior=ee.enum.switches.breakerBehavior.zeroCrossingEnable
      settings: InternalSimscapePortConfiguration="{\"Bottom\":[],\"Left\":[{\"id\":\"vT\",\"label\":\"vT\",\"type\":\"input\"},{\"id\":\"N1\",\"label\":\"~1\",\"type\":\"foundation.electrical.three_phase\"}],\"Right\":[{\"id\":\"N2\",\"label\":\"~2\",\"type\":\"foundation.electrical.three_phase\"}],\"Top\":[]}"
  Conn1 : PMIOPort  Side=Right
  Conn2 : PMIOPort  Port=2  Side=Left
  Conn3 : PMIOPort  Port=3  Side=Left
  connections:
  Conn1/RConn1 -- Circuit Breaker at GEN2/RConn1
  Circuit Breaker at GEN2/LConn1 -- Conn3/RConn1
  Circuit Breaker at GEN2/LConn2 -- Conn2/RConn1

== system Cyber_Physical_Microgrid/Subsystem2 ==
  Circuit Breaker at GEN3 : ee_lib/Switches & Breakers/Circuit Breaker (Three-Phase)  R_closed=1e-6 Ohm  G_open=1e-6 1/Ohm  threshold=0.5 V  breaker_behavior=ee.enum.switches.breakerBehavior.zeroCrossingEnable
      settings: InternalSimscapePortConfiguration="{\"Bottom\":[],\"Left\":[{\"id\":\"vT\",\"label\":\"vT\",\"type\":\"input\"},{\"id\":\"N1\",\"label\":\"~1\",\"type\":\"foundation.electrical.three_phase\"}],\"Right\":[{\"id\":\"N2\",\"label\":\"~2\",\"type\":\"foundation.electrical.three_phase\"}],\"Top\":[]}"
  Conn1 : PMIOPort  Side=Right
  Conn2 : PMIOPort  Port=2  Side=Left
  Conn3 : PMIOPort  Port=3  Side=Left
  connections:
  Circuit Breaker at GEN3/LConn2 -- Conn3/RConn1
  Conn1/RConn1 -- Circuit Breaker at GEN3/RConn1
  Conn2/RConn1 -- Circuit Breaker at GEN3/LConn1

== system Cyber_Physical_Microgrid/Subsystem3 ==
  Circuit Breaker at GEN4 : ee_lib/Switches & Breakers/Circuit Breaker (Three-Phase)  R_closed=1e-6 Ohm  G_open=1e-6 1/Ohm  threshold=0.5 V  breaker_behavior=ee.enum.switches.breakerBehavior.zeroCrossingEnable
      settings: InternalSimscapePortConfiguration="{\"Bottom\":[],\"Left\":[{\"id\":\"vT\",\"label\":\"vT\",\"type\":\"input\"},{\"id\":\"N1\",\"label\":\"~1\",\"type\":\"foundation.electrical.three_phase\"}],\"Right\":[{\"id\":\"N2\",\"label\":\"~2\",\"type\":\"foundation.electrical.three_phase\"}],\"Top\":[]}"
  Conn1 : PMIOPort  Side=Right
  Conn2 : PMIOPort  Port=2  Side=Left
  Conn3 : PMIOPort  Port=3  Side=Left
  connections:
  Conn3/RConn1 -- Circuit Breaker at GEN4/LConn1
  Conn2/RConn1 -- Circuit Breaker at GEN4/LConn2
  Circuit Breaker at GEN4/RConn1 -- Conn1/RConn1

== system Cyber_Physical_Microgrid/Subsystem4 ==
  Circuit Breaker : ee_lib/Switches & Breakers/Circuit Breaker  R_closed=0.001 Ohm  G_open=1e-6 1/Ohm  threshold=0.5 V  breaker_behavior=ee.enum.switches.breakerBehavior.zeroCrossingDisable
      settings: InternalSimscapePortConfiguration="{\"Bottom\":[],\"Left\":[{\"id\":\"vT\",\"label\":\"vT\",\"type\":\"input\"},{\"id\":\"p1\",\"label\":\"\",\"type\":\"foundation.electrical.electrical\"}],\"Right\":[{\"id\":\"p2\",\"label\":\"\",\"type\":\"foundation.electrical.electrical\"}],\"Top\":[]}"
  Conn1 : PMIOPort  Side=Right
  Conn2 : PMIOPort  Port=2  Side=Left
  Conn3 : PMIOPort  Port=3  Side=Left
  connections:
  Circuit Breaker/RConn1 -- Conn1/RConn1
  Conn2/RConn1 -- Circuit Breaker/LConn1
  Circuit Breaker/LConn2 -- Conn3/RConn1

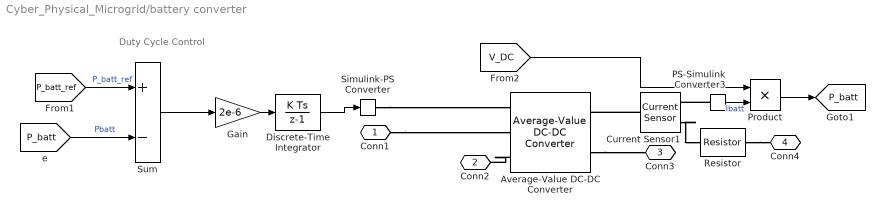
== system Cyber_Physical_Microgrid/battery converter ==
  note: Duty Cycle Control
  Average-Value DC-DC Converter : ee_lib/Semiconductors & Converters/Converters/Average-Value DC-DC Converter  control_option=ee.enum.converters.controlinput.dutycycle  converter_type=ee.enum.converters.dcdctype.buckboost  efficiency_option=ee.enum.converters.efficiency.constant  efficiency_fixed=100  i_vec=[0, 2, 5] A  efficiency_vec=[90, 95, 98]
      settings: InternalSimscapePortConfiguration="{\"Bottom\":[],\"Left\":[{\"id\":\"DutyCycle\",\"label\":\"DutyCycle\",\"type\":\"input\"},{\"id\":\"p1\",\"label\":\"1+\",\"type\":\"foundation.electrical.electrical\"},{\"id\":\"n1\",\"label\":\"1-\",\"type\":\"foundation.electrical.electrical\"}],\"Right\":[{\"id\":\"p2\",\"label\":\"2+\",\"type\":\"foundation.electrical.electrical\"},{\"id\":\"n2\",\"label\":\"2-\",\"type\":\"foundation.electrical.electrical\"}],\"Top\":[]}"
  Current Sensor1 : fl_lib/Electrical/Electrical Sensors/Current Sensor
  Discrete-Time Integrator : DiscreteIntegrator  InitialCondition=0.5  SampleTime=Ts_DC  LimitOutput=on  UpperSaturationLimit=0.99  LowerSaturationLimit=0  ICPrevOutput=DiscIntNeverNeededParam  ICPrevScaledInput=DiscIntNeverNeededParam
  Gain : Gain  Gain=2e-6
  PS-Simulink Converter3 : nesl_utility/PS-Simulink Converter  PhysicalDomain=network_engine_domain  SubClassName=ps_output  LeftPortType=input  RightPortType=output  PseudoPeriodic=off  Frequencies=[]  VectorFormat=1-D array  Unit=inherit  AffineConversion=off
  Product : Product
  Resistor : fl_lib/Electrical/Electrical Elements/Resistor  R=1e-3 Ohm  i_specify=off  i_priority=None  i=0 A  i_nominal_specify=off  i_nominal_value=1  i_nominal_unit=A  v_specify=off  v_priority=None  v=0 V  v_nominal_specify=off  v_nominal_value=1  v_nominal_unit=V
  Simulink-PS Converter : nesl_utility/Simulink-PS Converter  PhysicalDomain=network_engine_domain  SubClassName=ps_input  LeftPortType=input  RightPortType=output  PseudoPeriodic=off  Frequencies=[]  NoiseDistribution=none  NoiseParameters=[]  Unit=1  AffineConversion=off  FilteringAndDerivatives=provide  SimscapeFilterOrder=1  InputFilterTimeConstant=0.001  UdotUserProvided=0
  Sum : Sum  Inputs=+-
  Conn1 : PMIOPort  Side=Left
  Conn2 : PMIOPort  Port=2  Side=Left
  Conn3 : PMIOPort  Port=3  Side=Right
  Conn4 : PMIOPort  Port=4  Side=Right
  tag scope: P_batt=global
  wires:
  PS-Simulink Converter3/1 -> Product/2  "Ibatt"
  Discrete-Time Integrator/1 -> Simulink-PS Converter/1
  Product/1 -> [P_batt]
  [P_batt] -> Sum/2  "Pbatt"
  [V_DC] -> Product/1
  [P_batt_ref] -> Sum/1  "P_batt_ref"
  Gain/1 -> Discrete-Time Integrator/1
  Sum/1 -> Gain/1
  connections:
  Average-Value DC-DC Converter/LConn3 -- Conn2/RConn1
  Current Sensor1/RConn2 -- Resistor/LConn1
  Conn1/RConn1 -- Average-Value DC-DC Converter/LConn2
  PS-Simulink Converter3/LConn1 -- Current Sensor1/RConn1
  Current Sensor1/LConn1 -- Average-Value DC-DC Converter/RConn1
  Simulink-PS Converter/RConn1 -- Average-Value DC-DC Converter/LConn1
  Resistor/RConn1 -- Conn4/RConn1
  Average-Value DC-DC Converter/RConn2 -- Conn3/RConn1

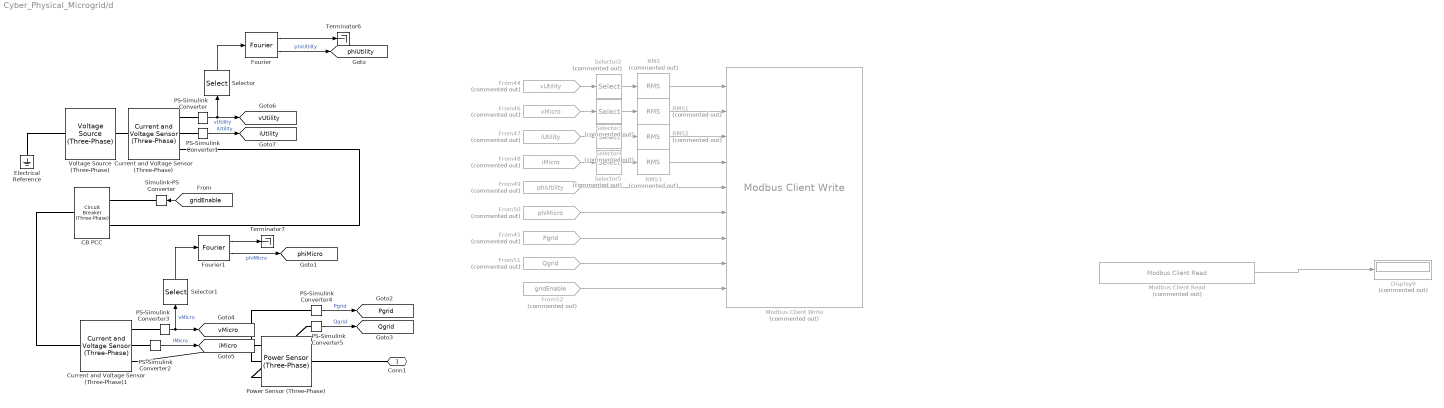
== system Cyber_Physical_Microgrid/d ==
  CB PCC : ee_lib/Switches & Breakers/Circuit Breaker (Three-Phase)  R_closed=1e-6 Ohm  G_open=1e-6 1/Ohm  threshold=0.5 V  breaker_behavior=ee.enum.switches.breakerBehavior.zeroCrossingEnable
      settings: InternalSimscapePortConfiguration="{\"Bottom\":[],\"Left\":[{\"id\":\"vT\",\"label\":\"vT\",\"type\":\"input\"},{\"id\":\"N1\",\"label\":\"~1\",\"type\":\"foundation.electrical.three_phase\"}],\"Right\":[{\"id\":\"N2\",\"label\":\"~2\",\"type\":\"foundation.electrical.three_phase\"}],\"Top\":[]}"
  Current and Voltage Sensor (Three-Phase) : ee_lib/Sensors & Transducers/Current and Voltage Sensor (Three-Phase)  vMeasurementType=ee.enum.vmeasurement.lg  outputUnit=ee.enum.unit.si  SRated=100e6 A*V  VRated=24e3 V  I_specify=off  I_priority=None  I=[0, 0, 0] A  I_nominal_specify=off  I_nominal_value=1  I_nominal_unit=A  V_specify=off  V_priority=None  V=[0, 0, 0] V  V_nominal_specify=off  V_nominal_value=1  V_nominal_unit=V
      settings: InternalSimscapePortConfiguration="{\"Bottom\":[],\"Left\":[{\"id\":\"N1\",\"label\":\"~1\",\"type\":\"foundation.electrical.three_phase\"}],\"Right\":[{\"id\":\"V_output\",\"label\":\"V\",\"type\":\"output\"},{\"id\":\"I_output\",\"label\":\"I\",\"type\":\"output\"},{\"id\":\"N2\",\"label\":\"~2\",\"type\":\"foundation.electrical.three_phase\"}],\"Top\":[]}"
  Current and Voltage Sensor (Three-Phase)1 : ee_lib/Sensors & Transducers/Current and Voltage Sensor (Three-Phase)  vMeasurementType=ee.enum.vmeasurement.lg  outputUnit=ee.enum.unit.si  SRated=100e6 A*V  VRated=24e3 V  I_specify=off  I_priority=None  I=[0, 0, 0] A  I_nominal_specify=off  I_nominal_value=1  I_nominal_unit=A  V_specify=off  V_priority=None  V=[0, 0, 0] V  V_nominal_specify=off  V_nominal_value=1  V_nominal_unit=V
      settings: InternalSimscapePortConfiguration="{\"Bottom\":[],\"Left\":[{\"id\":\"N1\",\"label\":\"~1\",\"type\":\"foundation.electrical.three_phase\"}],\"Right\":[{\"id\":\"V_output\",\"label\":\"V\",\"type\":\"output\"},{\"id\":\"I_output\",\"label\":\"I\",\"type\":\"output\"},{\"id\":\"N2\",\"label\":\"~2\",\"type\":\"foundation.electrical.three_phase\"}],\"Top\":[]}"
  Display9 : Display  Commented=on
  Electrical Reference : fl_lib/Electrical/Electrical Elements/Electrical Reference
  Fourier : spsFourierLib/Fourier  Freq=50  n=1  InInit=[0, 0]  Ts=Ts_AC
  Fourier1 : spsFourierLib/Fourier  Freq=50  n=1  InInit=[0, 0]  Ts=Ts_AC
  From44 : From  Commented=on  GotoTag=vUtility  TagVisibility=global
  From45 : From  Commented=on  GotoTag=Pgrid  TagVisibility=global
  From46 : From  Commented=on  GotoTag=vMicro  TagVisibility=global
  From47 : From  Commented=on  GotoTag=iUtility  TagVisibility=global
  From48 : From  Commented=on  GotoTag=iMicro  TagVisibility=global
  From49 : From  Commented=on  GotoTag=phiUtility  TagVisibility=global
  From50 : From  Commented=on  GotoTag=phiMicro  TagVisibility=global
  From51 : From  Commented=on  GotoTag=Qgrid  TagVisibility=global
  From52 : From  Commented=on  GotoTag=gridEnable  TagVisibility=global
  Modbus Client Read : modbuslib/Modbus Client Read  Commented=on  RetainClient=No Modbus client available  ClientList=No Modbus client available  ConnectionEndpoint=No Modbus client selected  ServerId=1  RegisterTable={ '1', 'synchStart', '38', 'Coil', 'bit', '1' }  SampleTime=1
  Modbus Client Write : modbuslib/Modbus Client Write  Commented=on  RetainClient=No Modbus client available  ClientList=No Modbus client available  ConnectionEndpoint=No Modbus client selected  ServerId=1  RegisterTable={ '1', 'vUtility_rms', '1', 'Holding Register', 'double'; '2', 'vMicro_rms', '5', 'Holding Register', 'double'; '3', 'iUtility_rms', '9', 'Holding Register', 'double'; '4', 'iMicro_rms', '13', 'Holding Register', 'double'; '5', 'phiUtility', '17', 'Holding Register', 'double'; '6', 'phiMicro', '21', 'Holding Register', 'double'; '7', 'Pgrid', '25', 'Holding Register', 'double'; '8', 'Qgrid', '29', 'Holding Register', 'double'; '9', 'gridEnable', '34', 'Coil', 'bit' }  SampleTime=1
  PS-Simulink Converter{,1..5} (6 alike) : nesl_utility/PS-Simulink Converter  PhysicalDomain=network_engine_domain  SubClassName=ps_output  LeftPortType=input  RightPortType=output  PseudoPeriodic=off  Frequencies=[]  VectorFormat=inherit  Unit=inherit  AffineConversion=off
  Power Sensor (Three-Phase) : ee_lib/Sensors & Transducers/Power Sensor (Three-Phase)  load_type=ee.enum.passive.type_balanced.balanced  f0=50 Hz
      settings: InternalSimscapePortConfiguration="{\"Bottom\":[],\"Left\":[{\"id\":\"N1\",\"label\":\"~1\",\"type\":\"foundation.electrical.three_phase\"}],\"Right\":[{\"id\":\"N2\",\"label\":\"~2\",\"type\":\"foundation.electrical.three_phase\"}],\"Top\":[{\"id\":\"Pm\",\"label\":\"P\",\"type\":\"output\"},{\"id\":\"Qm\",\"label\":\"Q\",\"type\":\"output\"}]}"
  RMS{,1..3} (4 alike) : spsRMSLib/RMS  Commented=on  TrueRMS=on  Freq=50  RMSInit=120  Ts=0
  Selector : Selector  InputPortWidth=3  IndexOptions=Index vector (dialog)  Indices=1  OutputSizes=1
  Selector1 : Selector  InputPortWidth=3  IndexOptions=Index vector (dialog)  Indices=1  OutputSizes=1
  Selector{2..5} (4 alike) : Selector  Commented=on  InputPortWidth=3  IndexOptions=Index vector (dialog)  Indices=1  OutputSizes=1
  Simulink-PS Converter : nesl_utility/Simulink-PS Converter  PhysicalDomain=network_engine_domain  SubClassName=ps_input  LeftPortType=input  RightPortType=output  PseudoPeriodic=off  Frequencies=[]  NoiseDistribution=none  NoiseParameters=[]  Unit=1  AffineConversion=off  FilteringAndDerivatives=provide  SimscapeFilterOrder=1  InputFilterTimeConstant=0.001  UdotUserProvided=0
  Terminator6 : Terminator
  Terminator7 : Terminator
  Voltage Source (Three-Phase) : ee_lib/Sources/Voltage Source (Three-Phase)  vline_rms=6600 V  shift=0 deg  freq=50 Hz  impedance_option=0  SShortCircuit=1e6 A*V  XR=15  R=0.01 Ohm  L=3.97e-4 H  harmonic_option=0  harmonic_orders=[5, 7, 11, 13]  harmonic_ratios=[.1, .1, .1, .1]  G_parasitic=0 1/Ohm  I_specify=off  I_priority=None  I=[0, 0, 0] A  I_nominal_specify=off  I_nominal_value=1  I_nominal_unit=A
  Conn1 : PMIOPort  Side=Right
  tag scope: Pgrid=global, Qgrid=global, iMicro=global, iUtility=global, phiMicro=global, phiUtility=global, vMicro=global, vUtility=global
  wires:
  PS-Simulink Converter5/1 -> [Qgrid]  "Qgrid"
  PS-Simulink Converter2/1 -> [iMicro]  "iMicro"
  Fourier1/1 -> Terminator7/1
  Fourier/1 -> Terminator6/1
  Fourier1/2 -> [phiMicro]  "phiMicro"
  Selector/1 -> Fourier/1
  Selector1/1 -> Fourier1/1
  PS-Simulink Converter4/1 -> [Pgrid]  "Pgrid"
  Fourier/2 -> [phiUtility]  "phiUtility"
  PS-Simulink Converter/1 -> [vUtility], Selector/1  "vUtility"
  PS-Simulink Converter1/1 -> [iUtility]  "iUtility"
  PS-Simulink Converter3/1 -> [vMicro], Selector1/1  "vMicro"
  Modbus Client Read/1 -> Display9/1
  From49/1 -> Modbus Client Write/5
  From52/1 -> Modbus Client Write/9
  RMS2/1 -> Modbus Client Write/3
  Selector4/1 -> RMS2/1
  From46/1 -> Selector3/1
  From50/1 -> Modbus Client Write/6
  RMS3/1 -> Modbus Client Write/4
  RMS1/1 -> Modbus Client Write/2
  From48/1 -> Selector5/1
  From51/1 -> Modbus Client Write/8
  Selector2/1 -> RMS/1
  RMS/1 -> Modbus Client Write/1
  Selector5/1 -> RMS3/1
  From44/1 -> Selector2/1
  From47/1 -> Selector4/1
  Selector3/1 -> RMS1/1
  From45/1 -> Modbus Client Write/7
  [gridEnable] -> Simulink-PS Converter/1
  connections:
  Power Sensor (Three-Phase)/LConn3 -- PS-Simulink Converter5/LConn1
  Current and Voltage Sensor (Three-Phase)/RConn3 -- CB PCC/LConn2
  PS-Simulink Converter/LConn1 -- Current and Voltage Sensor (Three-Phase)/RConn1
  Power Sensor (Three-Phase)/LConn1 -- Current and Voltage Sensor (Three-Phase)1/RConn3
  Current and Voltage Sensor (Three-Phase)1/LConn1 -- CB PCC/RConn1
  Electrical Reference/LConn1 -- Voltage Source (Three-Phase)/LConn1
  Conn1/RConn1 -- Power Sensor (Three-Phase)/RConn1
  PS-Simulink Converter2/LConn1 -- Current and Voltage Sensor (Three-Phase)1/RConn2
  PS-Simulink Converter1/LConn1 -- Current and Voltage Sensor (Three-Phase)/RConn2
  Power Sensor (Three-Phase)/LConn2 -- PS-Simulink Converter4/LConn1
  PS-Simulink Converter3/LConn1 -- Current and Voltage Sensor (Three-Phase)1/RConn1
  Current and Voltage Sensor (Three-Phase)/LConn1 -- Voltage Source (Three-Phase)/RConn1
  CB PCC/LConn1 -- Simulink-PS Converter/RConn1

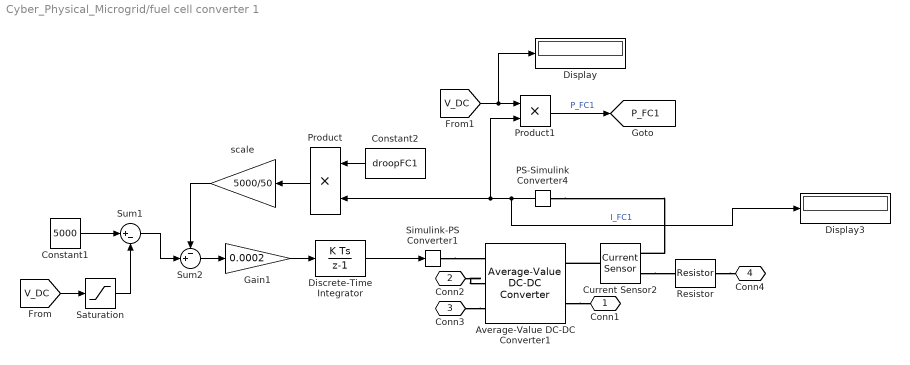
== system Cyber_Physical_Microgrid/fuel cell converter 1 ==
  Average-Value DC-DC Converter1 : ee_lib/Semiconductors & Converters/Converters/Average-Value DC-DC Converter  control_option=ee.enum.converters.controlinput.dutycycle  converter_type=ee.enum.converters.dcdctype.buckboost  efficiency_option=ee.enum.converters.efficiency.constant  efficiency_fixed=100  i_vec=[0, 2, 5] A  efficiency_vec=[90, 95, 98]
      settings: InternalSimscapePortConfiguration="{\"Bottom\":[],\"Left\":[{\"id\":\"DutyCycle\",\"label\":\"DutyCycle\",\"type\":\"input\"},{\"id\":\"p1\",\"label\":\"1+\",\"type\":\"foundation.electrical.electrical\"},{\"id\":\"n1\",\"label\":\"1-\",\"type\":\"foundation.electrical.electrical\"}],\"Right\":[{\"id\":\"p2\",\"label\":\"2+\",\"type\":\"foundation.electrical.electrical\"},{\"id\":\"n2\",\"label\":\"2-\",\"type\":\"foundation.electrical.electrical\"}],\"Top\":[]}"
  Constant1 : Constant  Value=5000  SampleTime=Ts_DC
  Constant2 : Constant  Value=droopFC1  SampleTime=Ts_DC
  Current Sensor2 : fl_lib/Electrical/Electrical Sensors/Current Sensor
  Discrete-Time Integrator : DiscreteIntegrator  gainval=1  InitialCondition=0.5  SampleTime=Ts_DC  LimitOutput=on  UpperSaturationLimit=0.99  LowerSaturationLimit=0  ICPrevOutput=DiscIntNeverNeededParam  ICPrevScaledInput=DiscIntNeverNeededParam
  Display : Display
  Display3 : Display
  Gain1 : Gain  Gain=0.0002
  PS-Simulink Converter4 : nesl_utility/PS-Simulink Converter  PhysicalDomain=network_engine_domain  SubClassName=ps_output  LeftPortType=input  RightPortType=output  PseudoPeriodic=off  Frequencies=[]  VectorFormat=1-D array  Unit=inherit  AffineConversion=off
  Product : Product
  Product1 : Product
  Resistor : fl_lib/Electrical/Electrical Elements/Resistor  R=1e-3 Ohm  i_specify=off  i_priority=None  i=0 A  i_nominal_specify=off  i_nominal_value=1  i_nominal_unit=A  v_specify=off  v_priority=None  v=0 V  v_nominal_specify=off  v_nominal_value=1  v_nominal_unit=V
  Saturation : Saturate  UpperLimit=5000
  Simulink-PS Converter1 : nesl_utility/Simulink-PS Converter  PhysicalDomain=network_engine_domain  SubClassName=ps_input  LeftPortType=input  RightPortType=output  PseudoPeriodic=off  Frequencies=[]  NoiseDistribution=none  NoiseParameters=[]  Unit=1  AffineConversion=off  FilteringAndDerivatives=provide  SimscapeFilterOrder=1  InputFilterTimeConstant=0.001  UdotUserProvided=0
  Sum1 : Sum  Inputs=|+-
  Sum2 : Sum  Inputs=-+|
  scale : Gain  Gain=5000/50
  Conn1 : PMIOPort  Side=Right
  Conn2 : PMIOPort  Port=2  Side=Left
  Conn3 : PMIOPort  Port=3  Side=Left
  Conn4 : PMIOPort  Port=4  Side=Right
  tag scope: P_FC1=global
  wires:
  Product/1 -> scale/1
  Sum2/1 -> Gain1/1
  Sum1/1 -> Sum2/2
  Product1/1 -> [P_FC1]  "P_FC1"
  Gain1/1 -> Discrete-Time Integrator/1
  [V_DC] -> Saturation/1
  Saturation/1 -> Sum1/2
  [V_DC] -> Display/1, Product1/1
  Constant2/1 -> Product/1
  PS-Simulink Converter4/1 -> Display3/1, Product/2, Product1/2  "I_FC1"
  Discrete-Time Integrator/1 -> Simulink-PS Converter1/1
  Constant1/1 -> Sum1/1
  scale/1 -> Sum2/1
  connections:
  Current Sensor2/RConn2 -- Resistor/LConn1
  Simulink-PS Converter1/RConn1 -- Average-Value DC-DC Converter1/LConn1
  Average-Value DC-DC Converter1/RConn2 -- Conn1/RConn1
  Conn3/RConn1 -- Average-Value DC-DC Converter1/LConn3
  PS-Simulink Converter4/LConn1 -- Current Sensor2/RConn1
  Current Sensor2/LConn1 -- Average-Value DC-DC Converter1/RConn1
  Resistor/RConn1 -- Conn4/RConn1
  Conn2/RConn1 -- Average-Value DC-DC Converter1/LConn2
